simulink model "ex7p3"  (R2016b)
settings: Solver=VariableStepAuto  StartTime=0.0  StopTime=0.5  RelTol=1e-3
libraries: powerlib x12, powerlib_meascontrol x5
settings Model: Creator=user  LastModifiedBy=user

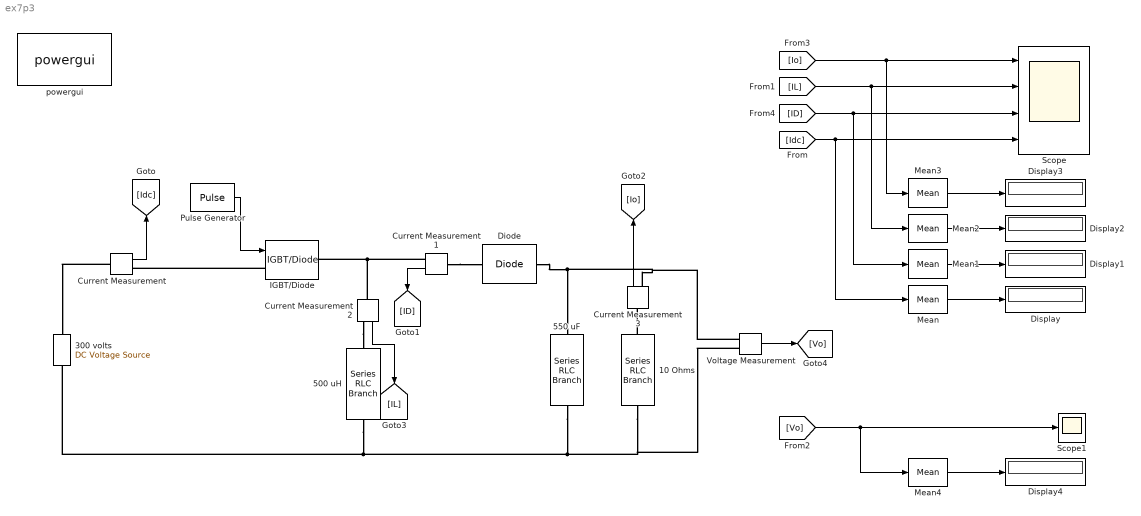
== system ex7p3 ==
  10 Ohms : powerlib/Elements/Series RLC Branch  LConnTagsString=__new0  RConnTagsString=__new0  BranchType=R  Resistance=10  Inductance=1e-3  SetiL0=off  InitialCurrent=0  Capacitance=1e-6  Setx0=off  InitialVoltage=0  Measurements=None
  300 volts : powerlib/Electrical Sources/DC Voltage Source  Amplitude=300  Measurements=None
  500 uH : powerlib/Elements/Series RLC Branch  LConnTagsString=__new0  RConnTagsString=__new0  BranchType=L  Resistance=1  Inductance=500e-6  SetiL0=off  InitialCurrent=0  Capacitance=1e-6  Setx0=off  InitialVoltage=0  Measurements=None
  550 uF : powerlib/Elements/Series RLC Branch  LConnTagsString=__new0  RConnTagsString=__new0  BranchType=C  Resistance=1  Inductance=1e-3  SetiL0=off  InitialCurrent=0  Capacitance=550e-6  Setx0=on  InitialVoltage=150  Measurements=None
  Current Measurement{,1..3} (4 alike) : powerlib/Measurements/Current Measurement  PhasorSimulation=off  OutputType=Complex  PSBequivalent=0
  Diode : powerlib/Power Electronics/Diode  Ron=0.001  Lon=0  Vf=0.8  IC=0  UseSnubber=off  Rs=0  Cs=0  Measurements=off
  Display{,1..4} (5 alike) : Display
  IGBT/Diode : powerlib/Power Electronics/IGBT//Diode  Ron=1e-3  Rs=1e5  Cs=inf  Measurements=off
  Mean{,1..4} (5 alike) : powerlib_meascontrol/Measurements/Mean  Freq=60  Vinit=0  Ts=0
  Pulse Generator : DiscretePulseGenerator  PulseType=Time based  Period=1/10000  PulseWidth=90
  Scope : Scope  NumInputPorts=4
  Scope1 : Scope
  Voltage Measurement : powerlib/Measurements/Voltage Measurement  PhasorSimulation=off  OutputType=Complex  PSBequivalent=0
  powergui : powerlib/powergui  Priority=1  SimulationMode=Continuous  SolverType=Tustin/Backward Euler (TBE)  SampleTime=50e-6  frequency=60  SPID=off  DisableSnubberDevices=off  DisableRonSwitches=off  DisableVfSwitches=off  SwTol=0  DisplayEquations=off  Interpol=off  ExternalGateDelay=off  methode=off  Ts=10  FunctionMessages=off  echomessages=off  HookPort=off  EnableUseOfTLC=off  x0status=blocks  frequencyindice=0  Pbase=100e6  ErrMax=1e-4  Iterations=50  UnitsV=kV  UnitsW=MW  buscounter=0  RestoreLinks=warning  ResistiveCurrentMeasurement=off  Frange=[0:2:500]  Ylog=off  Xlog=on  ShowGrid=off  save=off  variable=ZData  structure=0  ZoomFFT=off  StartTime=0.0  cycles=1  DisplayStyle=1  fundamental=60  FreqAxis=off  MaxFrequency=1000  frequencyindicesteady=1  RmsSteady=1  display=off
  wires:
  Pulse Generator/1 -> IGBT/Diode/1
  Current Measurement2/1 -> [IL]
  Current Measurement/1 -> [Idc]
  Voltage Measurement/1 -> [Vo]
  [Vo] -> Mean4/1, Scope1/1
  Mean4/1 -> Display4/1
  [Idc] -> Scope/4, Mean/1
  [ID] -> Scope/3, Mean1/1
  [IL] -> Scope/2, Mean2/1
  [Io] -> Scope/1, Mean3/1
  Mean3/1 -> Display3/1
  Mean2/1 -> Display2/1
  Mean/1 -> Display/1
  Mean1/1 -> Display1/1
  Current Measurement1/1 -> [ID]
  Current Measurement3/1 -> [Io]
  connections:
  550 uF/RConn1 -- Voltage Measurement/LConn1 -- 10 Ohms/RConn1 -- 500 uH/RConn1 -- 300 volts/LConn1
  Diode/LConn1 -- Voltage Measurement/LConn2 -- Current Measurement3/RConn1 -- 550 uF/LConn1
  Current Measurement/LConn1 -- 300 volts/RConn1
  IGBT/Diode/LConn1 -- Current Measurement/RConn1
  Current Measurement2/RConn1 -- 500 uH/LConn1
  Current Measurement2/LConn1 -- Current Measurement1/RConn1 -- IGBT/Diode/RConn1
  Current Measurement1/LConn1 -- Diode/RConn1
  10 Ohms/LConn1 -- Current Measurement3/LConn1
